simulink model "OBSTACLE_DETECTION"  (R2023a)
settings: Solver=FixedStepDiscrete  StartTime=0.0  StopTime=10.0  FixedStep=0.01  RelTol=1e-3
undefined symbols (not defined in the file or in its folder): InputPWM, WheelSpeed
libraries: mobileRoboticsTrainingLib x5
settings Model: Creator=nuvitdemirtas  LastModifiedBy=nuvitdemirtas

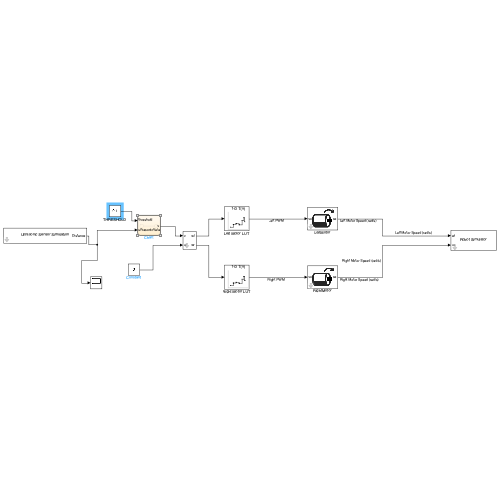
[thumbnail: Simulink's stored preview of the top-level diagram]
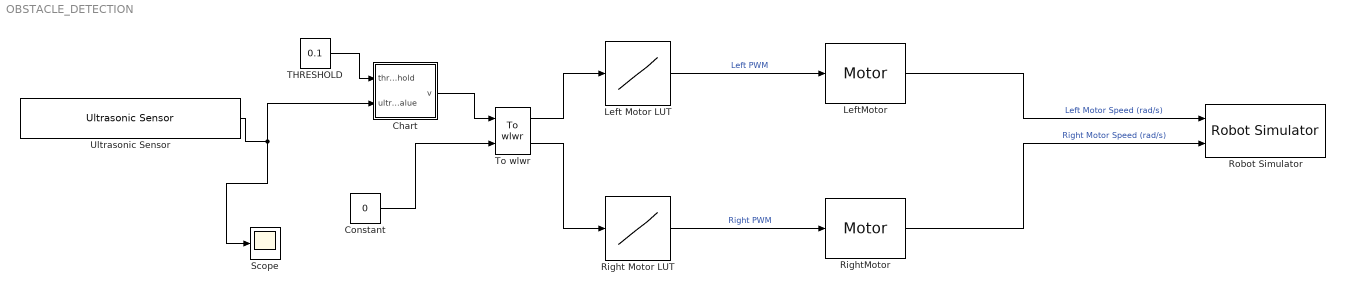
== system OBSTACLE_DETECTION ==
  Chart : Stateflow chart  TreatAsAtomicUnit=on
  Constant : Constant  Value=0
  Left Motor LUT : Lookup_n-D  NumberOfTableDimensions=1  BreakpointsForDimension1=WheelSpeed  Table=InputPWM  InterpMethod=Nearest  ExtrapMethod=Clip  InternalRulePriority=Speed  RndMeth=Simplest
  LeftMotor : mobileRoboticsTrainingLib/Motor  motorPlant=wheelMotorModel  sensorType=Speed
      settings: SourceProductName=Mobile Robotics Training Library
  Right Motor LUT : Lookup_n-D  NumberOfTableDimensions=1  BreakpointsForDimension1=WheelSpeed  Table=InputPWM  InterpMethod=Nearest  ExtrapMethod=Clip  InternalRulePriority=Speed  RndMeth=Simplest
  RightMotor : mobileRoboticsTrainingLib/Motor  motorPlant=wheelMotorModel  sensorType=Speed
      settings: SourceProductName=Mobile Robotics Training Library
  Robot Simulator : mobileRoboticsTrainingLib/Robot Simulator  Priority=99  mapVar=mapForSim  startX=5.2776  startY=4.9821  startTheta=0  axleLength=axleLength  wheelR=wheelR
  Scope : Scope
  THRESHOLD : Constant  Value=0.1
  To wlwr : mobileRoboticsTrainingLib/To wlwr  axleLength=0.1  wheelR=0.05
  Ultrasonic Sensor : mobileRoboticsTrainingLib/Ultrasonic Sensor  mapVar=mapForSim  maxSenRange=4  minSenRange=0.02  senRes=0.003  sensOff=[0.1 0]
      settings: SourceProductName=Mobile Robotics Training Library
  wires:
  Right Motor LUT/1 -> RightMotor/1  "Right PWM"
  RightMotor/1 -> Robot Simulator/2  "Right Motor Speed (rad/s)"
  To wlwr/1 -> Left Motor LUT/1
  Left Motor LUT/1 -> LeftMotor/1  "Left PWM"
  LeftMotor/1 -> Robot Simulator/1  "Left Motor Speed (rad/s)"
  To wlwr/2 -> Right Motor LUT/1
  Constant/1 -> To wlwr/2
  Ultrasonic Sensor/1 -> Scope/1, Chart/2(ultrasonicValue)
  THRESHOLD/1 -> Chart/1(threshold)
  Chart/1(v) -> To wlwr/1

== stateflow chart OBSTACLE_DETECTION/Chart ==
  state GoForward
    entry: v = 0.2
  state Stop
    entry: v = 0
  (default) -> GoForward
  Stop -> GoForward : [ultrasonicValue > threshold]
  GoForward -> Stop : [ultrasonicValue <= threshold]
  data: threshold input; ultrasonicValue input; v output
